simulink model "General_model_Step2_NonMinimal"  (R2020b)
settings: Solver=VariableStepAuto  StartTime=0.0  StopTime=10.0  RelTol=1e-3
libraries: RCTblocks x1
settings Model: Creator=pa.iannelli  LastModifiedBy=f.sanfedino

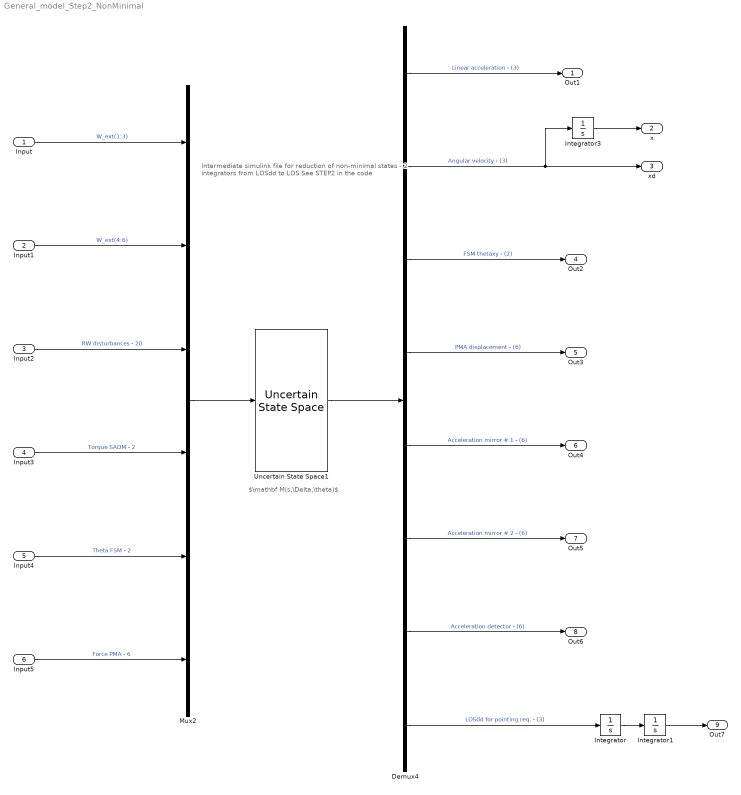
== system General_model_Step2_NonMinimal ==
  note: Intermediate simulink file for reduction of non-minimal states
      |
      | - 2 integrators from LOSdd to LOS
      |
      | See STEP2 in the code
  note: $\mathbf M(s,\Delta,\theta)$
  Input : Inport
  Input1 : Inport  Port=2
  Input2 : Inport  Port=3
  Input3 : Inport  Port=4
  Input4 : Inport  Port=5
  Input5 : Inport  Port=6
  Demux4 : Demux  Outputs=[3 3,2,6,6,6,6,3]
  Integrator : Integrator
  Integrator1 : Integrator
  Integrator3 : Integrator
  Mux2 : Mux  Inputs=[3,3,20,2,2,6]
  Uncertain State Space1 : RCTblocks/Uncertain State Space  Tag=USS  SCDEnableBlockLinearizationSpecification=on  USystem=Gum_IOselected_AfterStep1  UValue=[]  X0=[]  uX0=[]
      settings: SourceProductBaseCode=RC
  Out1 : Outport
  x : Outport  Port=2
  xd : Outport  Port=3
  Out2 : Outport  Port=4
  Out3 : Outport  Port=5
  Out4 : Outport  Port=6
  Out5 : Outport  Port=7
  Out6 : Outport  Port=8
  Out7 : Outport  Port=9
  wires:
  Uncertain State Space1/1 -> Demux4/1
  Mux2/1 -> Uncertain State Space1/1
  Demux4/8 -> Integrator/1  "LOSdd for pointing req. - (3)"
  Demux4/1 -> Out1/1  "Linear acceleration - (3)"
  Demux4/2 -> xd/1, Integrator3/1  "Angular velocity - (3)"
  Integrator3/1 -> x/1
  Integrator/1 -> Integrator1/1
  Demux4/3 -> Out2/1  "FSM thetaxy - (2)"
  Demux4/4 -> Out3/1  "PMA displacement - (6)"
  Demux4/5 -> Out4/1  "Acceleration mirror # 1 - (6)"
  Demux4/6 -> Out5/1  "Acceleration mirror # 2 - (6)"
  Demux4/7 -> Out6/1  "Acceleration detector - (6)"
  Integrator1/1 -> Out7/1
  Input/1 -> Mux2/1  "W_ext(1:3)"
  Input1/1 -> Mux2/2  "W_ext(4:6)"
  Input2/1 -> Mux2/3  "RW disturbances - 20"
  Input3/1 -> Mux2/4  "Torque SADM - 2"
  Input4/1 -> Mux2/5  "Theta FSM - 2"
  Input5/1 -> Mux2/6  "Force PMA - 6"
